simulink model "ClosedLoopModels"  (R2018a)
settings: Solver=VariableStepAuto  StartTime=0.0  StopTime=10  RelTol=1e-3
values from neighbouring files (symbols this model uses):
  dfdi = 0.0422490961327    [LinearizedN=50.mat]    (also in SystemClosedLoopControl.m = 0.0793; SystemPositionSweep.m = (netForce_current(linearizationPointIndex+2)-netForce_curren; linearizationRun.mat)
  dfdz = -0.115865440563    [LinearizedN=50.mat]    (also in SystemClosedLoopControl.m = -0.0877; SystemPositionSweep.m = (netZForce(linearizationPointIndex+2)-netZForce(linearizatio; linearizationRun.mat)
  M = 0.0068    [SystemClosedLoopControl.m]
libraries: simulink x2
settings Model: Creator=Tom  LastModifiedBy=Tom

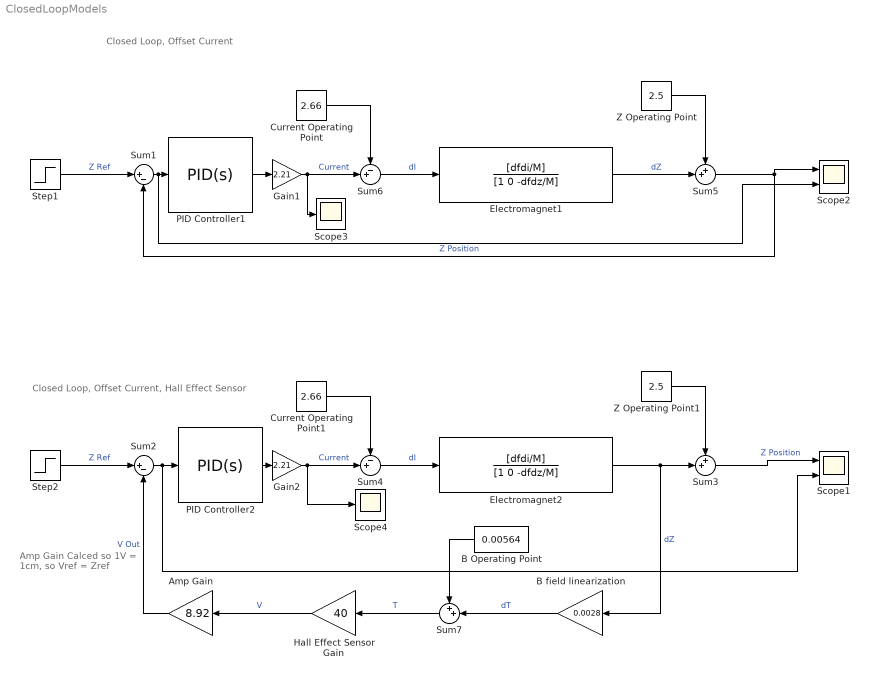
== system ClosedLoopModels ==
  note: Amp Gain Calced so 1V = 1cm,
      | so Vref = Zref
  note: Closed Loop, Offset Current
  note: Closed Loop, Offset Current, Hall Effect Sensor
  Amp Gain : Gain  Gain=8.92
  B Operating Point : Constant  Value=0.00564
  B field linearization : Gain  Gain=0.0028
  Current Operating Point : Constant  Value=2.66
  Current Operating Point1 : Constant  Value=2.66
  Electromagnet1 : TransferFcn  Numerator=[dfdi/M]  Denominator=[1 0 -dfdz/M]
  Electromagnet2 : TransferFcn  Numerator=[dfdi/M]  Denominator=[1 0 -dfdz/M]
  Gain1 : Gain  Gain=2.21
  Gain2 : Gain  Gain=2.21
  Hall Effect Sensor Gain : Gain  Gain=40
  PID Controller1 : simulink/Continuous/PID Controller  Controller=PID  TimeDomain=Continuous-time  SampleTime=-1  IntegratorMethod=Forward Euler  FilterMethod=Forward Euler  Form=Parallel  UseFilter=on  ControllerParametersSource=internal  P=1  I=1  D=1  N=100  InitialConditionSource=internal  InitialConditionForIntegrator=0  InitialConditionForFilter=0  ExternalReset=none  LimitOutput=on  UpperSaturationLimit=2.66/2.21  LowerSaturationLimit=-2.66/2.21  LinearizeAsGain=on  AntiWindupMode=none  Kb=1  TrackingMode=off  Kt=1  PParamMin=[]  PParamMax=[]  IParamMin=[]  IParamMax=[]  DParamMin=[]  DParamMax=[]  NParamMin=[]  NParamMax=[]  KbParamMin=[]  KbParamMax=[]  KtParamMin=[]  KtParamMax=[]  POutMin=[]  POutMax=[]  IOutMin=[]  IOutMax=[]  DOutMin=[]  DOutMax=[]  NOutMin=[]  NOutMax=[]  KbOutMin=[]  KbOutMax=[]  KtOutMin=[]  KtOutMax=[]  IntegratorOutMin=[]  IntegratorOutMax=[]  FilterOutMin=[]  FilterOutMax=[]  SumOutMin=[]  SumOutMax=[]  SumI1OutMin=[]  SumI1OutMax=[]  SumI2OutMin=[]  SumI2OutMax=[]  SumI3OutMin=[]  SumI3OutMax=[]  SumDOutMin=[]  SumDOutMax=[]  SaturationOutMin=[]  SaturationOutMax=[]  IntegratorContinuousStateAttributes=''  IntegratorStateMustResolveToSignalObject=off  IntegratorRTWStateStorageClass=Auto  FilterContinuousStateAttributes=''  FilterStateMustResolveToSignalObject=off  FilterRTWStateStorageClass=Auto  DifferentiatorICPrevScaledInput=0  DifferentiatorOutMin=[]  DifferentiatorOutMax=[]  FilterDiffOutCoefMin=[]  FilterDiffOutCoefMax=[]  SumDenOutMin=[]  SumDenOutMax=[]  SumNumOutMin=[]  SumNumOutMax=[]  ReciprocalOutMin=[]  ReciprocalOutMax=[]  DivideOutMin=[]  DivideOutMax=[]  TunerSelectOption=Frequency Response Based
  PID Controller2 : simulink/Continuous/PID Controller  Controller=PID  TimeDomain=Continuous-time  SampleTime=-1  IntegratorMethod=Forward Euler  FilterMethod=Forward Euler  Form=Parallel  UseFilter=on  ControllerParametersSource=internal  P=1  I=1  D=1  N=100  InitialConditionSource=internal  InitialConditionForIntegrator=0  InitialConditionForFilter=0  ExternalReset=none  LimitOutput=on  UpperSaturationLimit=2.66/2.21  LowerSaturationLimit=-2.66/2.21  LinearizeAsGain=on  AntiWindupMode=none  Kb=1  TrackingMode=off  Kt=1  PParamMin=[]  PParamMax=[]  IParamMin=[]  IParamMax=[]  DParamMin=[]  DParamMax=[]  NParamMin=[]  NParamMax=[]  KbParamMin=[]  KbParamMax=[]  KtParamMin=[]  KtParamMax=[]  POutMin=[]  POutMax=[]  IOutMin=[]  IOutMax=[]  DOutMin=[]  DOutMax=[]  NOutMin=[]  NOutMax=[]  KbOutMin=[]  KbOutMax=[]  KtOutMin=[]  KtOutMax=[]  IntegratorOutMin=[]  IntegratorOutMax=[]  FilterOutMin=[]  FilterOutMax=[]  SumOutMin=[]  SumOutMax=[]  SumI1OutMin=[]  SumI1OutMax=[]  SumI2OutMin=[]  SumI2OutMax=[]  SumI3OutMin=[]  SumI3OutMax=[]  SumDOutMin=[]  SumDOutMax=[]  SaturationOutMin=[]  SaturationOutMax=[]  IntegratorContinuousStateAttributes=''  IntegratorStateMustResolveToSignalObject=off  IntegratorRTWStateStorageClass=Auto  FilterContinuousStateAttributes=''  FilterStateMustResolveToSignalObject=off  FilterRTWStateStorageClass=Auto  DifferentiatorICPrevScaledInput=0  DifferentiatorOutMin=[]  DifferentiatorOutMax=[]  FilterDiffOutCoefMin=[]  FilterDiffOutCoefMax=[]  SumDenOutMin=[]  SumDenOutMax=[]  SumNumOutMin=[]  SumNumOutMax=[]  ReciprocalOutMin=[]  ReciprocalOutMax=[]  DivideOutMin=[]  DivideOutMax=[]  TunerSelectOption=Frequency Response Based
  Scope1 : Scope  NumInputPorts=2
  Scope2 : Scope  NumInputPorts=2
  Scope3 : Scope
  Scope4 : Scope
  Step1 : Step  Time=0  After=2.5  SampleTime=0
  Step2 : Step  Time=0  After=2.5  SampleTime=0
  Sum1 : Sum  Inputs=|+-
  Sum2 : Sum  Inputs=|+-
  Sum3 : Sum  Inputs=++|
  Sum4 : Sum  Inputs=-+|
  Sum5 : Sum  Inputs=++|
  Sum6 : Sum  Inputs=-+|
  Sum7 : Sum  Inputs=++|
  Z Operating Point : Constant  Value=2.5
  Z Operating Point1 : Constant  Value=2.5
  wires:
  Step1/1 -> Sum1/1  "Z Ref"
  Sum1/1 -> Scope2/2, PID Controller1/1
  PID Controller1/1 -> Gain1/1
  Sum5/1 -> Scope2/1, Sum1/2  "Z Position"
  Electromagnet1/1 -> Sum5/2  "dZ"
  Z Operating Point/1 -> Sum5/1
  Sum6/1 -> Electromagnet1/1  "dI"
  Gain1/1 -> Scope3/1, Sum6/2  "Current"
  Current Operating Point/1 -> Sum6/1
  Sum4/1 -> Electromagnet2/1  "dI"
  Current Operating Point1/1 -> Sum4/1
  Step2/1 -> Sum2/1  "Z Ref"
  Sum3/1 -> Scope1/1  "Z Position"
  Gain2/1 -> Scope4/1, Sum4/2  "Current"
  Electromagnet2/1 -> B field linearization/1, Sum3/2  "dZ"
  Z Operating Point1/1 -> Sum3/1
  PID Controller2/1 -> Gain2/1
  Sum2/1 -> Scope1/2, PID Controller2/1
  B field linearization/1 -> Sum7/2  "dT"
  Sum7/1 -> Hall Effect Sensor Gain/1  "T"
  B Operating Point/1 -> Sum7/1
  Hall Effect Sensor Gain/1 -> Amp Gain/1  "V"
  Amp Gain/1 -> Sum2/2  "V Out"
